simulink model "fxpdemo_dbl2fix"  (Simulink 5.0)
settings: Solver=FixedStepDiscrete  SolverMode=SingleTasking  StartTime=0.0  StopTime=1  FixedStep=0.001  RelTol=1e-3  AbsTol=1e-6
InitFcn:
  | ;fxptdlg('fxptdlg_simInit_cb');
StartFcn:
  | ;fxptdlg('fxptdlg_sim_cb');
StopFcn:
  | ;fxptdlg('fxptdlg_store_cb');
libraries: fixpt_lib_4 x2, fixpt_lib_3p1 x1
PreSaveFcn:
  | ;fxptdlg('fxptdlg_presave_cb');
CloseFcn:
  | ;fxptdlg('fxptdlg_close_cb');
settings Model: RequirementInfo=9  CovMetricSettings=d  DataTypeOverride=ForceOff  MinMaxOverflowLogging=MinMaxAndOverflow  Creator=andyb  LastModifiedBy=andyb  ExtModeTrigMode=oneshot  ExtModeArmWhenConnect=off  ExtModeAutoUpdateStatusClock=off  LimitDataPoints=off  IntegerOverflowMsg=none  ParameterDowncastMsg=warning  ParameterOverflowMsg=warning  ParameterPrecisionLossMsg=none  BooleanDataType=off

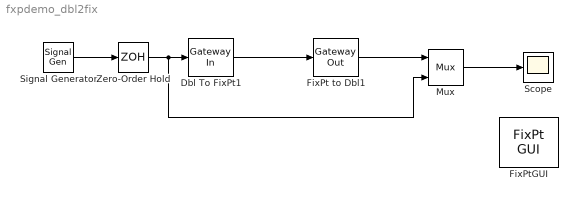
== system fxpdemo_dbl2fix ==
  Dbl To FixPt1 : fixpt_lib_4/Data Type/Gateway In  InRealWorld=Real World Value  OutputDataTypeScalingMode=Specify via dialog  OutDataType=sfix(5)  OutScaling=2^-2  DoSatur=off
  FixPt to Dbl1 : fixpt_lib_4/Data Type/Gateway Out  OutRealWorld=Real World Value  OutBuiltInType=double  DoSatur=off
  FixPtGUI : fixpt_lib_3p1/FixPt GUI
  Mux : Mux  Inputs=2
  Scope : Scope
      settings: TickLabels=on  TimeRange=1  YMin=-10  YMax=10
  Signal Generator : SignalGenerator  WaveForm=sawtooth  Amplitude=10
  Zero-Order Hold : ZeroOrderHold  SampleTime=0.001
  wires:
  Zero-Order Hold/1 -> Dbl To FixPt1/1, Mux/2
  Signal Generator/1 -> Zero-Order Hold/1
  FixPt to Dbl1/1 -> Mux/1
  Dbl To FixPt1/1 -> FixPt to Dbl1/1
  Mux/1 -> Scope/1
